simulink model "sys_model"  (R2020b)
settings: Solver=VariableStepAuto  StartTime=0.0  StopTime=10  RelTol=1e-3
settings Model: Creator=Rasika Shejul  LastModifiedBy=Rushikesh

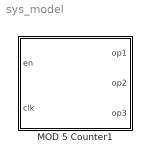
== system sys_model ==
  MOD 5 Counter1 : Stateflow chart  TreatAsAtomicUnit=on

== stateflow chart sys_model/MOD 5 Counter1 ==
  state State_1
    en:
    op1 = 0;
    op2 = 0;
    op3 = 0;
  state State_2
    en:
    op1 = 0;
    op2 = 0;
    op3 = 0;
  state State_8
    en:
    op1 = 0;
    op2 = 0;
    op3 = 0;
  state State_3
    en:
    op1 = 0;
    op2 = 0;
    op3 = 0;
  state State_7
    en:
    op1 = 0;
    op2 = 0;
    op3 = 0;
  state State_4
    en:
    op1 = 0;
    op2 = 0;
    op3 = 0;
  state State_6
    en:
    op1 = 0;
    op2 = 0;
    op3 = 0;
  state State_5
    en:
    op1 = 0;
    op2 = 0;
    op3 = 0;
  (default) -> State_1
  State_1 -> State_2 : [clk ==1]
  State_8 -> State_1 : [clk ==1]
  State_2 -> State_3 : [clk ==1]
  (junction 29) -> State_1 [order 1] : [en == 1]
  State_7 -> State_8 : [clk ==1]
  State_3 -> State_4 : [clk ==1]
  State_6 -> State_7 : [clk ==1]
  State_4 -> State_5 : [clk ==1]
  (junction 29) -> State_6 [order 2] : [en == 0]
  State_5 -> (junction 29) : [clk ==1]
  data: op1 output; op2 output; op3 output; en input; clk input
